simulink model "modelStab3"  (R2013b)
settings: Solver=ode4  StartTime=0.0  StopTime=tSim  FixedStep=h  RelTol=1e-3
values from neighbouring files (symbols this model uses):
  modelSelect = 'full'    [launcher_script.m]    (also in launcher_simulink.m = 'linear')
  params = [M,m,L,I,b,g]    [launcher_script.m]    (also in launcher_simulink.m)
  state0 = [thetaDot0;theta0;xDot0;x0]    [launcher_script.m]    (also in launcher_simulink.m; sFunction.m = [])
settings Model: Creator=JAR  LastModifiedBy=JAR

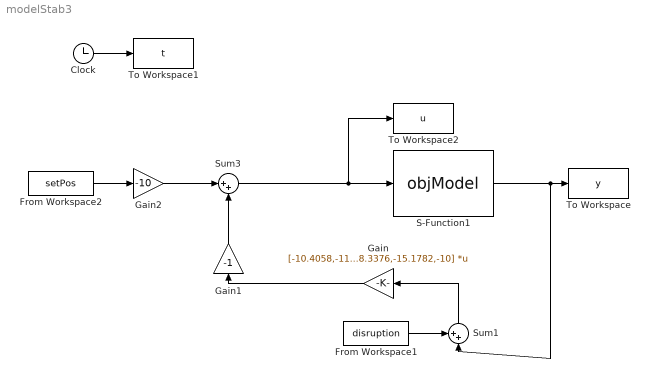
== system modelStab3 ==
  Clock : Clock
  From Workspace1 : FromWorkspace  VariableName=disruption  SampleTime=0
  From Workspace2 : FromWorkspace  VariableName=setPos  SampleTime=0
  Gain : Gain  Gain=[-10.4058,-118.3376,-15.1782,-10]  Multiplication=Matrix(K*u)
  Gain1 : Gain  Gain=-1
  Gain2 : Gain  Gain=-10
  S-Function1 : S-Function  FunctionName=objModel  Parameters=state0,params,modelSelect  EnableBusSupport=off
  Sum1 : Sum  Inputs=++|
  Sum3 : Sum  Inputs=|++
  To Workspace : ToWorkspace  VariableName=y  SampleTime=-1
  To Workspace1 : ToWorkspace  VariableName=t  SampleTime=-1
  To Workspace2 : ToWorkspace  VariableName=u  SampleTime=-1
  wires:
  Clock/1 -> To Workspace1/1
  S-Function1/1 -> Sum1/2, To Workspace/1
  Gain/1 -> Gain1/1
  From Workspace1/1 -> Sum1/1
  Sum1/1 -> Gain/1
  Gain1/1 -> Sum3/2
  From Workspace2/1 -> Gain2/1
  Gain2/1 -> Sum3/1
  Sum3/1 -> To Workspace2/1, S-Function1/1
